simulink model "TST_CrCtl_StTrans"  (R2016b)
settings: Solver=FixedStepDiscrete  StartTime=0.0  StopTime=simTime  FixedStep=sampleTime  RelTol=1e-3
values from neighbouring files (symbols this model uses):
  testCase = 1    [initTST_CrCtl_StTrans_001.m]    (also in initTST_CrCtl_StTrans_002.m = 2; initTST_CrCtl_StTrans_003.m = 3; initTST_CrCtl_StTrans_004.m = 4; initTST_CrCtl_StTrans_005.m = 5)
libraries: simulink x46, UnitTest_Lib x5
(part 2 of 2)

== system TST_CrCtl_StTrans/simulationInput/testSignals_R003 ==
  BC : BusCreator  Inputs=22
  spec_CrCUI_stBttn : FromWorkspace  VariableName=testSig_CrCUI_stBttn  Interpolate=off  OutputAfterFinalValue=Holding final value
  spec_CrCtl_rTraV2NBeg : FromWorkspace  VariableName=testSig_CrCtl_rTraV2NBeg  Interpolate=off  OutputAfterFinalValue=Holding final value
  spec_CrCtl_rTraV2NBeg_raw : FromWorkspace  VariableName=testSig_CrCtl_rTraV2NBeg_raw  Interpolate=off  OutputAfterFinalValue=Holding final value
  spec_CrCtl_st : FromWorkspace  VariableName=testSig_CrCtl_st  Interpolate=off  OutputAfterFinalValue=Holding final value
  spec_CrCtl_stAccSave : FromWorkspace  VariableName=testSig_CrCtl_stAccSave  Interpolate=off  OutputAfterFinalValue=Holding final value
  spec_CrCtl_stCrCUIvLimAdj : FromWorkspace  VariableName=testSig_CrCtl_stCrCUIvLimAdj  Interpolate=off  OutputAfterFinalValue=Holding final value
  spec_CrCtl_stDecSave : FromWorkspace  VariableName=testSig_CrCtl_stDecSave  Interpolate=off  OutputAfterFinalValue=Holding final value
  spec_CrCtl_stLck : FromWorkspace  VariableName=testSig_CrCtl_stLck  Interpolate=off  OutputAfterFinalValue=Holding final value
  spec_CrCtl_stOpFunc : FromWorkspace  VariableName=testSig_CrCtl_stOpFunc  Interpolate=off  OutputAfterFinalValue=Holding final value
  spec_CrCtl_stReq : FromWorkspace  VariableName=testSig_CrCtl_stReq  Interpolate=off  OutputAfterFinalValue=Holding final value
  spec_CrCtl_stShOff : FromWorkspace  VariableName=testSig_CrCtl_stShOff  Interpolate=off  OutputAfterFinalValue=Holding final value
  spec_CrCtl_stStTrans : FromWorkspace  VariableName=testSig_CrCtl_stStTrans  Interpolate=off  OutputAfterFinalValue=Holding final value
  spec_CrCtl_stSub : FromWorkspace  VariableName=testSig_CrCtl_stSub  Interpolate=off  OutputAfterFinalValue=Holding final value
  spec_CrCtl_stSub_raw : FromWorkspace  VariableName=testSig_CrCtl_stSub_raw  Interpolate=off  OutputAfterFinalValue=Holding final value
  spec_CrCtl_stSusp : FromWorkspace  VariableName=testSig_CrCtl_stSusp  Interpolate=off  OutputAfterFinalValue=Holding final value
  spec_CrCtl_stSuspAct : FromWorkspace  VariableName=testSig_CrCtl_stSuspAct  Interpolate=off  OutputAfterFinalValue=Holding final value
  spec_CrCtl_st_raw : FromWorkspace  VariableName=testSig_CrCtl_st_raw  Interpolate=off  OutputAfterFinalValue=Holding final value
  spec_CrCtl_vDes : FromWorkspace  VariableName=testSig_CrCtl_vDes  Interpolate=off  OutputAfterFinalValue=Holding final value
  spec_GlbDa_vXFlt : FromWorkspace  VariableName=testSig_GlbDa_vXFlt  Interpolate=off  OutputAfterFinalValue=Holding final value
  spec_LLim_stModify : FromWorkspace  VariableName=testSig_LLim_stModify  Interpolate=off  OutputAfterFinalValue=Holding final value
  spec_PT_rTraV2N : FromWorkspace  VariableName=testSig_PT_rTraV2N  Interpolate=off  OutputAfterFinalValue=Holding final value
  spec_WESDem_stCurr : FromWorkspace  VariableName=testSig_WESDem_stCurr  Interpolate=off  OutputAfterFinalValue=Holding final value
  testSignals : Outport
  wires:
  BC/1 -> testSignals/1
  spec_CrCtl_stLck/1 -> BC/1  "testSig_CrCtl_stLck"
  spec_CrCtl_stOpFunc/1 -> BC/2  "testSig_CrCtl_stOpFunc"
  spec_CrCtl_stReq/1 -> BC/3  "testSig_CrCtl_stReq"
  spec_CrCtl_stShOff/1 -> BC/4  "testSig_CrCtl_stShOff"
  spec_CrCtl_stSuspAct/1 -> BC/5  "testSig_CrCtl_stSuspAct"
  spec_CrCtl_vDes/1 -> BC/6  "testSig_CrCtl_vDes"
  spec_CrCUI_stBttn/1 -> BC/7  "testSig_CrCUI_stBttn"
  spec_GlbDa_vXFlt/1 -> BC/8  "testSig_GlbDa_vXFlt"
  spec_LLim_stModify/1 -> BC/9  "testSig_LLim_stModify"
  spec_PT_rTraV2N/1 -> BC/10  "testSig_PT_rTraV2N"
  spec_WESDem_stCurr/1 -> BC/11  "testSig_WESDem_stCurr"
  spec_CrCtl_st/1 -> BC/12  "testSig_CrCtl_st"
  spec_CrCtl_stSub/1 -> BC/13  "testSig_CrCtl_stSub"
  spec_CrCtl_rTraV2NBeg/1 -> BC/14  "testSig_CrCtl_rTraV2NBeg"
  spec_CrCtl_stAccSave/1 -> BC/15  "testSig_CrCtl_stAccSave"
  spec_CrCtl_stCrCUIvLimAdj/1 -> BC/16  "testSig_CrCtl_stCrCUIvLimAdj"
  spec_CrCtl_stDecSave/1 -> BC/17  "testSig_CrCtl_stDecSave"
  spec_CrCtl_stStTrans/1 -> BC/18  "testSig_CrCtl_stStTrans"
  spec_CrCtl_stSusp/1 -> BC/19  "testSig_CrCtl_stSusp"
  spec_CrCtl_rTraV2NBeg_raw/1 -> BC/20  "testSig_CrCtl_rTraV2NBeg_raw"
  spec_CrCtl_st_raw/1 -> BC/21  "testSig_CrCtl_st_raw"
  spec_CrCtl_stSub_raw/1 -> BC/22  "testSig_CrCtl_stSub_raw"

== system TST_CrCtl_StTrans/simulationInput/testSignals_R004 ==
  BC : BusCreator  Inputs=22
  spec_CrCUI_stBttn : FromWorkspace  VariableName=testSig_CrCUI_stBttn  Interpolate=off  OutputAfterFinalValue=Holding final value
  spec_CrCtl_rTraV2NBeg : FromWorkspace  VariableName=testSig_CrCtl_rTraV2NBeg  Interpolate=off  OutputAfterFinalValue=Holding final value
  spec_CrCtl_rTraV2NBeg_raw : FromWorkspace  VariableName=testSig_CrCtl_rTraV2NBeg_raw  Interpolate=off  OutputAfterFinalValue=Holding final value
  spec_CrCtl_st : FromWorkspace  VariableName=testSig_CrCtl_st  Interpolate=off  OutputAfterFinalValue=Holding final value
  spec_CrCtl_stAccSave : FromWorkspace  VariableName=testSig_CrCtl_stAccSave  Interpolate=off  OutputAfterFinalValue=Holding final value
  spec_CrCtl_stCrCUIvLimAdj : FromWorkspace  VariableName=testSig_CrCtl_stCrCUIvLimAdj  Interpolate=off  OutputAfterFinalValue=Holding final value
  spec_CrCtl_stDecSave : FromWorkspace  VariableName=testSig_CrCtl_stDecSave  Interpolate=off  OutputAfterFinalValue=Holding final value
  spec_CrCtl_stLck : FromWorkspace  VariableName=testSig_CrCtl_stLck  Interpolate=off  OutputAfterFinalValue=Holding final value
  spec_CrCtl_stOpFunc : FromWorkspace  VariableName=testSig_CrCtl_stOpFunc  Interpolate=off  OutputAfterFinalValue=Holding final value
  spec_CrCtl_stReq : FromWorkspace  VariableName=testSig_CrCtl_stReq  Interpolate=off  OutputAfterFinalValue=Holding final value
  spec_CrCtl_stShOff : FromWorkspace  VariableName=testSig_CrCtl_stShOff  Interpolate=off  OutputAfterFinalValue=Holding final value
  spec_CrCtl_stStTrans : FromWorkspace  VariableName=testSig_CrCtl_stStTrans  Interpolate=off  OutputAfterFinalValue=Holding final value
  spec_CrCtl_stSub : FromWorkspace  VariableName=testSig_CrCtl_stSub  Interpolate=off  OutputAfterFinalValue=Holding final value
  spec_CrCtl_stSub_raw : FromWorkspace  VariableName=testSig_CrCtl_stSub_raw  Interpolate=off  OutputAfterFinalValue=Holding final value
  spec_CrCtl_stSusp : FromWorkspace  VariableName=testSig_CrCtl_stSusp  Interpolate=off  OutputAfterFinalValue=Holding final value
  spec_CrCtl_stSuspAct : FromWorkspace  VariableName=testSig_CrCtl_stSuspAct  Interpolate=off  OutputAfterFinalValue=Holding final value
  spec_CrCtl_st_raw : FromWorkspace  VariableName=testSig_CrCtl_st_raw  Interpolate=off  OutputAfterFinalValue=Holding final value
  spec_CrCtl_vDes : FromWorkspace  VariableName=testSig_CrCtl_vDes  Interpolate=off  OutputAfterFinalValue=Holding final value
  spec_GlbDa_vXFlt : FromWorkspace  VariableName=testSig_GlbDa_vXFlt  Interpolate=off  OutputAfterFinalValue=Holding final value
  spec_LLim_stModify : FromWorkspace  VariableName=testSig_LLim_stModify  Interpolate=off  OutputAfterFinalValue=Holding final value
  spec_PT_rTraV2N : FromWorkspace  VariableName=testSig_PT_rTraV2N  Interpolate=off  OutputAfterFinalValue=Holding final value
  spec_WESDem_stCurr : FromWorkspace  VariableName=testSig_WESDem_stCurr  Interpolate=off  OutputAfterFinalValue=Holding final value
  testSignals : Outport
  wires:
  BC/1 -> testSignals/1
  spec_CrCtl_stLck/1 -> BC/1  "testSig_CrCtl_stLck"
  spec_CrCtl_stOpFunc/1 -> BC/2  "testSig_CrCtl_stOpFunc"
  spec_CrCtl_stReq/1 -> BC/3  "testSig_CrCtl_stReq"
  spec_CrCtl_stShOff/1 -> BC/4  "testSig_CrCtl_stShOff"
  spec_CrCtl_stSuspAct/1 -> BC/5  "testSig_CrCtl_stSuspAct"
  spec_CrCtl_vDes/1 -> BC/6  "testSig_CrCtl_vDes"
  spec_CrCUI_stBttn/1 -> BC/7  "testSig_CrCUI_stBttn"
  spec_GlbDa_vXFlt/1 -> BC/8  "testSig_GlbDa_vXFlt"
  spec_LLim_stModify/1 -> BC/9  "testSig_LLim_stModify"
  spec_PT_rTraV2N/1 -> BC/10  "testSig_PT_rTraV2N"
  spec_WESDem_stCurr/1 -> BC/11  "testSig_WESDem_stCurr"
  spec_CrCtl_st/1 -> BC/12  "testSig_CrCtl_st"
  spec_CrCtl_stSub/1 -> BC/13  "testSig_CrCtl_stSub"
  spec_CrCtl_rTraV2NBeg/1 -> BC/14  "testSig_CrCtl_rTraV2NBeg"
  spec_CrCtl_stAccSave/1 -> BC/15  "testSig_CrCtl_stAccSave"
  spec_CrCtl_stCrCUIvLimAdj/1 -> BC/16  "testSig_CrCtl_stCrCUIvLimAdj"
  spec_CrCtl_stDecSave/1 -> BC/17  "testSig_CrCtl_stDecSave"
  spec_CrCtl_stStTrans/1 -> BC/18  "testSig_CrCtl_stStTrans"
  spec_CrCtl_stSusp/1 -> BC/19  "testSig_CrCtl_stSusp"
  spec_CrCtl_rTraV2NBeg_raw/1 -> BC/20  "testSig_CrCtl_rTraV2NBeg_raw"
  spec_CrCtl_st_raw/1 -> BC/21  "testSig_CrCtl_st_raw"
  spec_CrCtl_stSub_raw/1 -> BC/22  "testSig_CrCtl_stSub_raw"

== system TST_CrCtl_StTrans/simulationInput/testSignals_R005 ==
  BC : BusCreator  Inputs=22
  spec_CrCUI_stBttn : FromWorkspace  VariableName=testSig_CrCUI_stBttn  Interpolate=off  OutputAfterFinalValue=Holding final value
  spec_CrCtl_rTraV2NBeg : FromWorkspace  VariableName=testSig_CrCtl_rTraV2NBeg  Interpolate=off  OutputAfterFinalValue=Holding final value
  spec_CrCtl_rTraV2NBeg_raw : FromWorkspace  VariableName=testSig_CrCtl_rTraV2NBeg_raw  Interpolate=off  OutputAfterFinalValue=Holding final value
  spec_CrCtl_st : FromWorkspace  VariableName=testSig_CrCtl_st  Interpolate=off  OutputAfterFinalValue=Holding final value
  spec_CrCtl_stAccSave : FromWorkspace  VariableName=testSig_CrCtl_stAccSave  Interpolate=off  OutputAfterFinalValue=Holding final value
  spec_CrCtl_stCrCUIvLimAdj : FromWorkspace  VariableName=testSig_CrCtl_stCrCUIvLimAdj  Interpolate=off  OutputAfterFinalValue=Holding final value
  spec_CrCtl_stDecSave : FromWorkspace  VariableName=testSig_CrCtl_stDecSave  Interpolate=off  OutputAfterFinalValue=Holding final value
  spec_CrCtl_stLck : FromWorkspace  VariableName=testSig_CrCtl_stLck  Interpolate=off  OutputAfterFinalValue=Holding final value
  spec_CrCtl_stOpFunc : FromWorkspace  VariableName=testSig_CrCtl_stOpFunc  Interpolate=off  OutputAfterFinalValue=Holding final value
  spec_CrCtl_stReq : FromWorkspace  VariableName=testSig_CrCtl_stReq  Interpolate=off  OutputAfterFinalValue=Holding final value
  spec_CrCtl_stShOff : FromWorkspace  VariableName=testSig_CrCtl_stShOff  Interpolate=off  OutputAfterFinalValue=Holding final value
  spec_CrCtl_stStTrans : FromWorkspace  VariableName=testSig_CrCtl_stStTrans  Interpolate=off  OutputAfterFinalValue=Holding final value
  spec_CrCtl_stSub : FromWorkspace  VariableName=testSig_CrCtl_stSub  Interpolate=off  OutputAfterFinalValue=Holding final value
  spec_CrCtl_stSub_raw : FromWorkspace  VariableName=testSig_CrCtl_stSub_raw  Interpolate=off  OutputAfterFinalValue=Holding final value
  spec_CrCtl_stSusp : FromWorkspace  VariableName=testSig_CrCtl_stSusp  Interpolate=off  OutputAfterFinalValue=Holding final value
  spec_CrCtl_stSuspAct : FromWorkspace  VariableName=testSig_CrCtl_stSuspAct  Interpolate=off  OutputAfterFinalValue=Holding final value
  spec_CrCtl_st_raw : FromWorkspace  VariableName=testSig_CrCtl_st_raw  Interpolate=off  OutputAfterFinalValue=Holding final value
  spec_CrCtl_vDes : FromWorkspace  VariableName=testSig_CrCtl_vDes  Interpolate=off  OutputAfterFinalValue=Holding final value
  spec_GlbDa_vXFlt : FromWorkspace  VariableName=testSig_GlbDa_vXFlt  Interpolate=off  OutputAfterFinalValue=Holding final value
  spec_LLim_stModify : FromWorkspace  VariableName=testSig_LLim_stModify  Interpolate=off  OutputAfterFinalValue=Holding final value
  spec_PT_rTraV2N : FromWorkspace  VariableName=testSig_PT_rTraV2N  Interpolate=off  OutputAfterFinalValue=Holding final value
  spec_WESDem_stCurr : FromWorkspace  VariableName=testSig_WESDem_stCurr  Interpolate=off  OutputAfterFinalValue=Holding final value
  testSignals : Outport
  wires:
  BC/1 -> testSignals/1
  spec_CrCtl_stLck/1 -> BC/1  "testSig_CrCtl_stLck"
  spec_CrCtl_stOpFunc/1 -> BC/2  "testSig_CrCtl_stOpFunc"
  spec_CrCtl_stReq/1 -> BC/3  "testSig_CrCtl_stReq"
  spec_CrCtl_stShOff/1 -> BC/4  "testSig_CrCtl_stShOff"
  spec_CrCtl_stSuspAct/1 -> BC/5  "testSig_CrCtl_stSuspAct"
  spec_CrCtl_vDes/1 -> BC/6  "testSig_CrCtl_vDes"
  spec_CrCUI_stBttn/1 -> BC/7  "testSig_CrCUI_stBttn"
  spec_GlbDa_vXFlt/1 -> BC/8  "testSig_GlbDa_vXFlt"
  spec_LLim_stModify/1 -> BC/9  "testSig_LLim_stModify"
  spec_PT_rTraV2N/1 -> BC/10  "testSig_PT_rTraV2N"
  spec_WESDem_stCurr/1 -> BC/11  "testSig_WESDem_stCurr"
  spec_CrCtl_st/1 -> BC/12  "testSig_CrCtl_st"
  spec_CrCtl_stSub/1 -> BC/13  "testSig_CrCtl_stSub"
  spec_CrCtl_rTraV2NBeg/1 -> BC/14  "testSig_CrCtl_rTraV2NBeg"
  spec_CrCtl_stAccSave/1 -> BC/15  "testSig_CrCtl_stAccSave"
  spec_CrCtl_stCrCUIvLimAdj/1 -> BC/16  "testSig_CrCtl_stCrCUIvLimAdj"
  spec_CrCtl_stDecSave/1 -> BC/17  "testSig_CrCtl_stDecSave"
  spec_CrCtl_stStTrans/1 -> BC/18  "testSig_CrCtl_stStTrans"
  spec_CrCtl_stSusp/1 -> BC/19  "testSig_CrCtl_stSusp"
  spec_CrCtl_rTraV2NBeg_raw/1 -> BC/20  "testSig_CrCtl_rTraV2NBeg_raw"
  spec_CrCtl_st_raw/1 -> BC/21  "testSig_CrCtl_st_raw"
  spec_CrCtl_stSub_raw/1 -> BC/22  "testSig_CrCtl_stSub_raw"

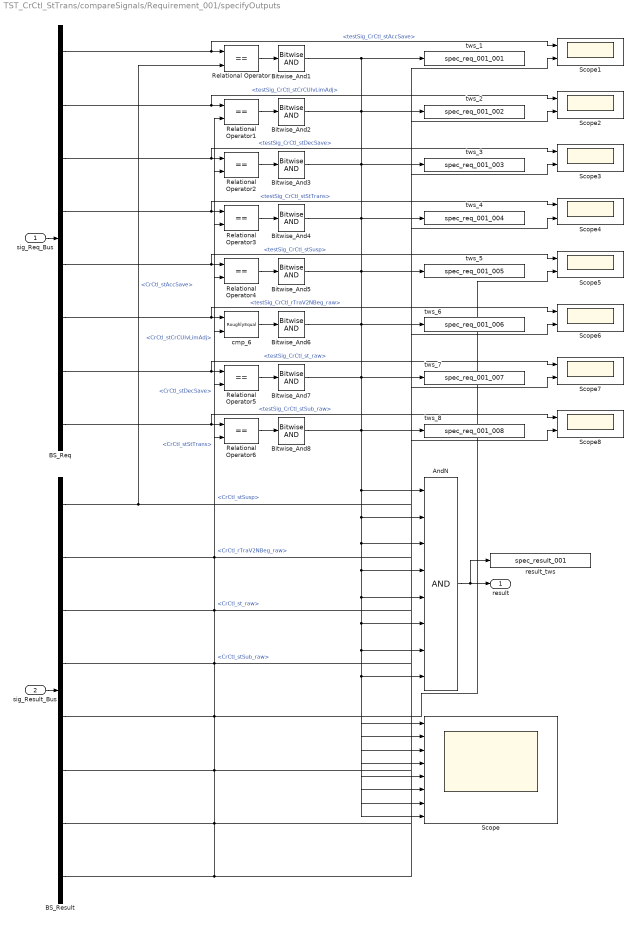
== system TST_CrCtl_StTrans/compareSignals/Requirement_001/specifyOutputs ==
  sig_Req_Bus : Inport
  sig_Result_Bus : Inport  Port=2
  AndN : Logic  Inputs=8
  BS_Req : BusSelector  OutputSignals=testSig_CrCtl_stAccSave,testSig_CrCtl_stCrCUIvLimAdj,testSig_CrCtl_stDecSave,testSig_CrCtl_stStTrans,testSig_CrCtl_stSusp,testSig_CrCtl_rTraV2NBeg_raw,testSig_CrCtl_st_raw,testSig_CrCtl_stSub_raw
  BS_Result : BusSelector  OutputSignals=CrCtl_stAccSave,CrCtl_stCrCUIvLimAdj,CrCtl_stDecSave,CrCtl_stStTrans,CrCtl_stSusp,CrCtl_rTraV2NBeg_raw,CrCtl_st_raw,CrCtl_stSub_raw
  Bitwise_And{1..8} (8 alike) : simulink/Logic and Bit Operations/Bitwise Operator  logicop=AND  UseBitMask=off  BitMask=bin2dec('11011001')  BitMaskRealWorld=Stored Integer
  Relational Operator{,1..6} (7 alike) : RelationalOperator  Operator===  OutDataTypeStr=boolean  RndMeth=Simplest
  Scope : Scope  NumInputPorts=8
  Scope{1..8} (8 alike) : Scope  NumInputPorts=2
  cmp_6 : UnitTest_Lib/RoughlyEqual  slope=0.1
  result_tws : ToWorkspace  VariableName=spec_result_001
  tws_1 : ToWorkspace  VariableName=spec_req_001_001
  tws_2 : ToWorkspace  VariableName=spec_req_001_002
  tws_3 : ToWorkspace  VariableName=spec_req_001_003
  tws_4 : ToWorkspace  VariableName=spec_req_001_004
  tws_5 : ToWorkspace  VariableName=spec_req_001_005
  tws_6 : ToWorkspace  VariableName=spec_req_001_006
  tws_7 : ToWorkspace  VariableName=spec_req_001_007
  tws_8 : ToWorkspace  VariableName=spec_req_001_008
  result : Outport
  wires:
  sig_Req_Bus/1 -> BS_Req/1
  sig_Result_Bus/1 -> BS_Result/1
  AndN/1 -> result/1, result_tws/1
  BS_Req/1 -> Relational Operator/1, Scope1/1  "<testSig_CrCtl_stAccSave>"
  BS_Result/1 -> Relational Operator/2, Scope1/2  "<CrCtl_stAccSave>"
  Relational Operator/1 -> Bitwise_And1/1
  Bitwise_And1/1 -> AndN/1, Scope/1, tws_1/1
  BS_Req/2 -> Relational Operator1/1, Scope2/1  "<testSig_CrCtl_stCrCUIvLimAdj>"
  BS_Result/2 -> Relational Operator1/2, Scope2/2  "<CrCtl_stCrCUIvLimAdj>"
  Relational Operator1/1 -> Bitwise_And2/1
  Bitwise_And2/1 -> AndN/2, Scope/2, tws_2/1
  BS_Req/3 -> Relational Operator2/1, Scope3/1  "<testSig_CrCtl_stDecSave>"
  BS_Result/3 -> Relational Operator2/2, Scope3/2  "<CrCtl_stDecSave>"
  Relational Operator2/1 -> Bitwise_And3/1
  Bitwise_And3/1 -> AndN/3, Scope/3, tws_3/1
  BS_Req/4 -> Relational Operator3/1, Scope4/1  "<testSig_CrCtl_stStTrans>"
  BS_Result/4 -> Relational Operator3/2, Scope4/2  "<CrCtl_stStTrans>"
  Relational Operator3/1 -> Bitwise_And4/1
  Bitwise_And4/1 -> AndN/4, Scope/4, tws_4/1
  BS_Req/5 -> Relational Operator4/1, Scope5/1  "<testSig_CrCtl_stSusp>"
  BS_Result/5 -> Relational Operator4/2, Scope5/2  "<CrCtl_stSusp>"
  Relational Operator4/1 -> Bitwise_And5/1
  Bitwise_And5/1 -> AndN/5, Scope/5, tws_5/1
  BS_Req/6 -> cmp_6/1, Scope6/1  "<testSig_CrCtl_rTraV2NBeg_raw>"
  BS_Result/6 -> cmp_6/2, Scope6/2  "<CrCtl_rTraV2NBeg_raw>"
  cmp_6/1 -> Bitwise_And6/1
  Bitwise_And6/1 -> AndN/6, Scope/6, tws_6/1
  BS_Req/7 -> Relational Operator5/1, Scope7/1  "<testSig_CrCtl_st_raw>"
  BS_Result/7 -> Relational Operator5/2, Scope7/2  "<CrCtl_st_raw>"
  Relational Operator5/1 -> Bitwise_And7/1
  Bitwise_And7/1 -> AndN/7, Scope/7, tws_7/1
  BS_Req/8 -> Relational Operator6/1, Scope8/1  "<testSig_CrCtl_stSub_raw>"
  BS_Result/8 -> Relational Operator6/2, Scope8/2  "<CrCtl_stSub_raw>"
  Relational Operator6/1 -> Bitwise_And8/1
  Bitwise_And8/1 -> AndN/8, Scope/8, tws_8/1

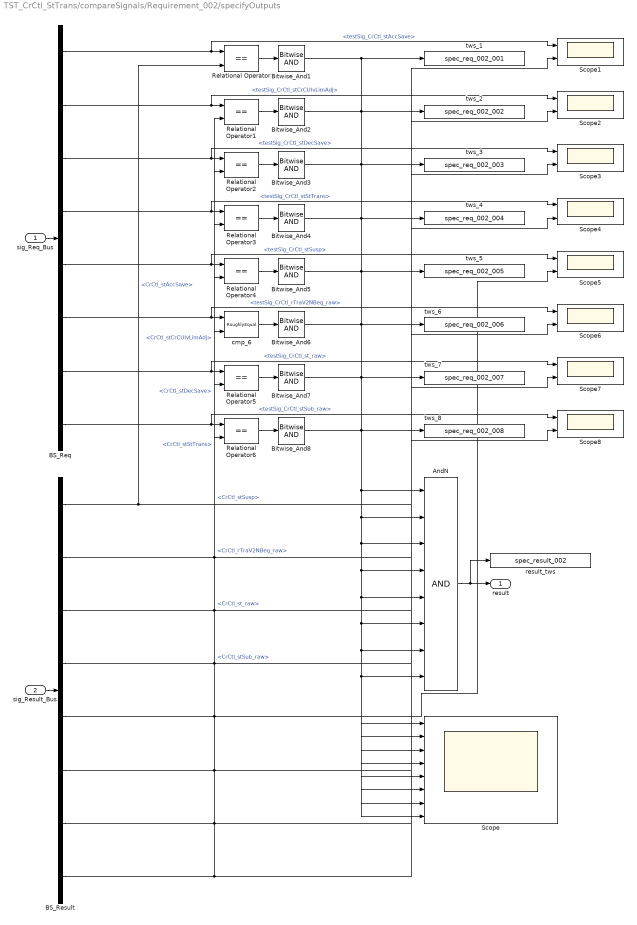
== system TST_CrCtl_StTrans/compareSignals/Requirement_002/specifyOutputs ==
  sig_Req_Bus : Inport
  sig_Result_Bus : Inport  Port=2
  AndN : Logic  Inputs=8
  BS_Req : BusSelector  OutputSignals=testSig_CrCtl_stAccSave,testSig_CrCtl_stCrCUIvLimAdj,testSig_CrCtl_stDecSave,testSig_CrCtl_stStTrans,testSig_CrCtl_stSusp,testSig_CrCtl_rTraV2NBeg_raw,testSig_CrCtl_st_raw,testSig_CrCtl_stSub_raw
  BS_Result : BusSelector  OutputSignals=CrCtl_stAccSave,CrCtl_stCrCUIvLimAdj,CrCtl_stDecSave,CrCtl_stStTrans,CrCtl_stSusp,CrCtl_rTraV2NBeg_raw,CrCtl_st_raw,CrCtl_stSub_raw
  Bitwise_And{1..8} (8 alike) : simulink/Logic and Bit Operations/Bitwise Operator  logicop=AND  UseBitMask=off  BitMask=bin2dec('11011001')  BitMaskRealWorld=Stored Integer
  Relational Operator{,1..6} (7 alike) : RelationalOperator  Operator===  OutDataTypeStr=boolean  RndMeth=Simplest
  Scope : Scope  NumInputPorts=8
  Scope{1..8} (8 alike) : Scope  NumInputPorts=2
  cmp_6 : UnitTest_Lib/RoughlyEqual  slope=0.1
  result_tws : ToWorkspace  VariableName=spec_result_002
  tws_1 : ToWorkspace  VariableName=spec_req_002_001
  tws_2 : ToWorkspace  VariableName=spec_req_002_002
  tws_3 : ToWorkspace  VariableName=spec_req_002_003
  tws_4 : ToWorkspace  VariableName=spec_req_002_004
  tws_5 : ToWorkspace  VariableName=spec_req_002_005
  tws_6 : ToWorkspace  VariableName=spec_req_002_006
  tws_7 : ToWorkspace  VariableName=spec_req_002_007
  tws_8 : ToWorkspace  VariableName=spec_req_002_008
  result : Outport
  wires:
  sig_Req_Bus/1 -> BS_Req/1
  sig_Result_Bus/1 -> BS_Result/1
  AndN/1 -> result/1, result_tws/1
  BS_Req/1 -> Relational Operator/1, Scope1/1  "<testSig_CrCtl_stAccSave>"
  BS_Result/1 -> Relational Operator/2, Scope1/2  "<CrCtl_stAccSave>"
  Relational Operator/1 -> Bitwise_And1/1
  Bitwise_And1/1 -> AndN/1, Scope/1, tws_1/1
  BS_Req/2 -> Relational Operator1/1, Scope2/1  "<testSig_CrCtl_stCrCUIvLimAdj>"
  BS_Result/2 -> Relational Operator1/2, Scope2/2  "<CrCtl_stCrCUIvLimAdj>"
  Relational Operator1/1 -> Bitwise_And2/1
  Bitwise_And2/1 -> AndN/2, Scope/2, tws_2/1
  BS_Req/3 -> Relational Operator2/1, Scope3/1  "<testSig_CrCtl_stDecSave>"
  BS_Result/3 -> Relational Operator2/2, Scope3/2  "<CrCtl_stDecSave>"
  Relational Operator2/1 -> Bitwise_And3/1
  Bitwise_And3/1 -> AndN/3, Scope/3, tws_3/1
  BS_Req/4 -> Relational Operator3/1, Scope4/1  "<testSig_CrCtl_stStTrans>"
  BS_Result/4 -> Relational Operator3/2, Scope4/2  "<CrCtl_stStTrans>"
  Relational Operator3/1 -> Bitwise_And4/1
  Bitwise_And4/1 -> AndN/4, Scope/4, tws_4/1
  BS_Req/5 -> Relational Operator4/1, Scope5/1  "<testSig_CrCtl_stSusp>"
  BS_Result/5 -> Relational Operator4/2, Scope5/2  "<CrCtl_stSusp>"
  Relational Operator4/1 -> Bitwise_And5/1
  Bitwise_And5/1 -> AndN/5, Scope/5, tws_5/1
  BS_Req/6 -> cmp_6/1, Scope6/1  "<testSig_CrCtl_rTraV2NBeg_raw>"
  BS_Result/6 -> cmp_6/2, Scope6/2  "<CrCtl_rTraV2NBeg_raw>"
  cmp_6/1 -> Bitwise_And6/1
  Bitwise_And6/1 -> AndN/6, Scope/6, tws_6/1
  BS_Req/7 -> Relational Operator5/1, Scope7/1  "<testSig_CrCtl_st_raw>"
  BS_Result/7 -> Relational Operator5/2, Scope7/2  "<CrCtl_st_raw>"
  Relational Operator5/1 -> Bitwise_And7/1
  Bitwise_And7/1 -> AndN/7, Scope/7, tws_7/1
  BS_Req/8 -> Relational Operator6/1, Scope8/1  "<testSig_CrCtl_stSub_raw>"
  BS_Result/8 -> Relational Operator6/2, Scope8/2  "<CrCtl_stSub_raw>"
  Relational Operator6/1 -> Bitwise_And8/1
  Bitwise_And8/1 -> AndN/8, Scope/8, tws_8/1

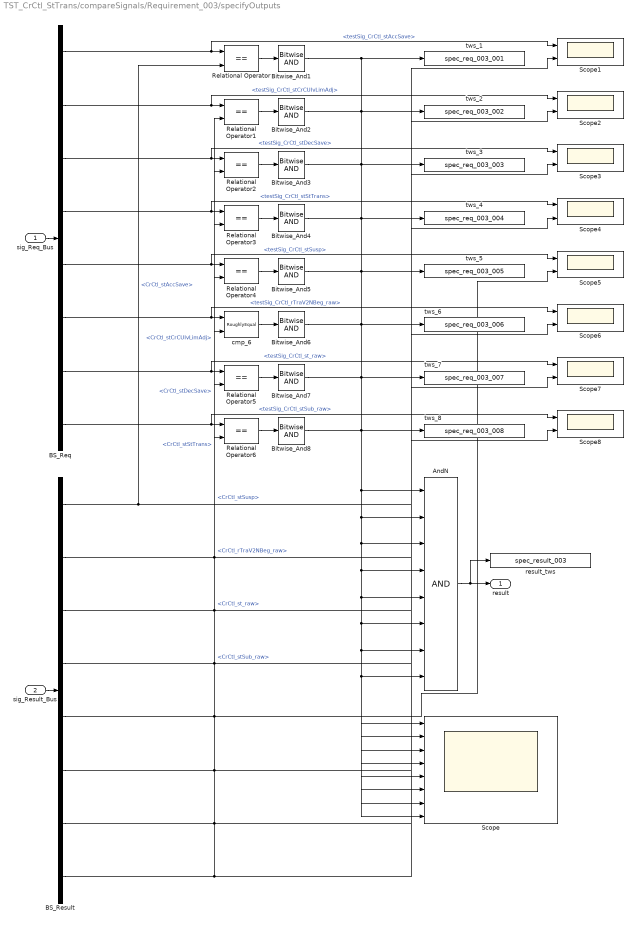
== system TST_CrCtl_StTrans/compareSignals/Requirement_003/specifyOutputs ==
  sig_Req_Bus : Inport
  sig_Result_Bus : Inport  Port=2
  AndN : Logic  Inputs=8
  BS_Req : BusSelector  OutputSignals=testSig_CrCtl_stAccSave,testSig_CrCtl_stCrCUIvLimAdj,testSig_CrCtl_stDecSave,testSig_CrCtl_stStTrans,testSig_CrCtl_stSusp,testSig_CrCtl_rTraV2NBeg_raw,testSig_CrCtl_st_raw,testSig_CrCtl_stSub_raw
  BS_Result : BusSelector  OutputSignals=CrCtl_stAccSave,CrCtl_stCrCUIvLimAdj,CrCtl_stDecSave,CrCtl_stStTrans,CrCtl_stSusp,CrCtl_rTraV2NBeg_raw,CrCtl_st_raw,CrCtl_stSub_raw
  Bitwise_And{1..8} (8 alike) : simulink/Logic and Bit Operations/Bitwise Operator  logicop=AND  UseBitMask=off  BitMask=bin2dec('11011001')  BitMaskRealWorld=Stored Integer
  Relational Operator{,1..6} (7 alike) : RelationalOperator  Operator===  OutDataTypeStr=boolean  RndMeth=Simplest
  Scope : Scope  NumInputPorts=8
  Scope{1..8} (8 alike) : Scope  NumInputPorts=2
  cmp_6 : UnitTest_Lib/RoughlyEqual  slope=0.1
  result_tws : ToWorkspace  VariableName=spec_result_003
  tws_1 : ToWorkspace  VariableName=spec_req_003_001
  tws_2 : ToWorkspace  VariableName=spec_req_003_002
  tws_3 : ToWorkspace  VariableName=spec_req_003_003
  tws_4 : ToWorkspace  VariableName=spec_req_003_004
  tws_5 : ToWorkspace  VariableName=spec_req_003_005
  tws_6 : ToWorkspace  VariableName=spec_req_003_006
  tws_7 : ToWorkspace  VariableName=spec_req_003_007
  tws_8 : ToWorkspace  VariableName=spec_req_003_008
  result : Outport
  wires:
  sig_Req_Bus/1 -> BS_Req/1
  sig_Result_Bus/1 -> BS_Result/1
  AndN/1 -> result/1, result_tws/1
  BS_Req/1 -> Relational Operator/1, Scope1/1  "<testSig_CrCtl_stAccSave>"
  BS_Result/1 -> Relational Operator/2, Scope1/2  "<CrCtl_stAccSave>"
  Relational Operator/1 -> Bitwise_And1/1
  Bitwise_And1/1 -> AndN/1, Scope/1, tws_1/1
  BS_Req/2 -> Relational Operator1/1, Scope2/1  "<testSig_CrCtl_stCrCUIvLimAdj>"
  BS_Result/2 -> Relational Operator1/2, Scope2/2  "<CrCtl_stCrCUIvLimAdj>"
  Relational Operator1/1 -> Bitwise_And2/1
  Bitwise_And2/1 -> AndN/2, Scope/2, tws_2/1
  BS_Req/3 -> Relational Operator2/1, Scope3/1  "<testSig_CrCtl_stDecSave>"
  BS_Result/3 -> Relational Operator2/2, Scope3/2  "<CrCtl_stDecSave>"
  Relational Operator2/1 -> Bitwise_And3/1
  Bitwise_And3/1 -> AndN/3, Scope/3, tws_3/1
  BS_Req/4 -> Relational Operator3/1, Scope4/1  "<testSig_CrCtl_stStTrans>"
  BS_Result/4 -> Relational Operator3/2, Scope4/2  "<CrCtl_stStTrans>"
  Relational Operator3/1 -> Bitwise_And4/1
  Bitwise_And4/1 -> AndN/4, Scope/4, tws_4/1
  BS_Req/5 -> Relational Operator4/1, Scope5/1  "<testSig_CrCtl_stSusp>"
  BS_Result/5 -> Relational Operator4/2, Scope5/2  "<CrCtl_stSusp>"
  Relational Operator4/1 -> Bitwise_And5/1
  Bitwise_And5/1 -> AndN/5, Scope/5, tws_5/1
  BS_Req/6 -> cmp_6/1, Scope6/1  "<testSig_CrCtl_rTraV2NBeg_raw>"
  BS_Result/6 -> cmp_6/2, Scope6/2  "<CrCtl_rTraV2NBeg_raw>"
  cmp_6/1 -> Bitwise_And6/1
  Bitwise_And6/1 -> AndN/6, Scope/6, tws_6/1
  BS_Req/7 -> Relational Operator5/1, Scope7/1  "<testSig_CrCtl_st_raw>"
  BS_Result/7 -> Relational Operator5/2, Scope7/2  "<CrCtl_st_raw>"
  Relational Operator5/1 -> Bitwise_And7/1
  Bitwise_And7/1 -> AndN/7, Scope/7, tws_7/1
  BS_Req/8 -> Relational Operator6/1, Scope8/1  "<testSig_CrCtl_stSub_raw>"
  BS_Result/8 -> Relational Operator6/2, Scope8/2  "<CrCtl_stSub_raw>"
  Relational Operator6/1 -> Bitwise_And8/1
  Bitwise_And8/1 -> AndN/8, Scope/8, tws_8/1

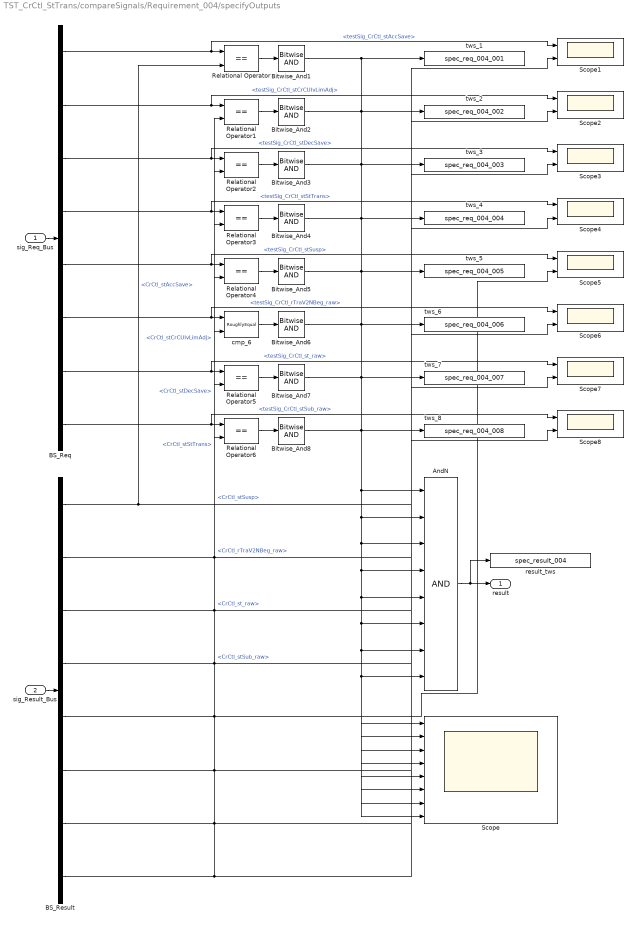
== system TST_CrCtl_StTrans/compareSignals/Requirement_004/specifyOutputs ==
  sig_Req_Bus : Inport
  sig_Result_Bus : Inport  Port=2
  AndN : Logic  Inputs=8
  BS_Req : BusSelector  OutputSignals=testSig_CrCtl_stAccSave,testSig_CrCtl_stCrCUIvLimAdj,testSig_CrCtl_stDecSave,testSig_CrCtl_stStTrans,testSig_CrCtl_stSusp,testSig_CrCtl_rTraV2NBeg_raw,testSig_CrCtl_st_raw,testSig_CrCtl_stSub_raw
  BS_Result : BusSelector  OutputSignals=CrCtl_stAccSave,CrCtl_stCrCUIvLimAdj,CrCtl_stDecSave,CrCtl_stStTrans,CrCtl_stSusp,CrCtl_rTraV2NBeg_raw,CrCtl_st_raw,CrCtl_stSub_raw
  Bitwise_And{1..8} (8 alike) : simulink/Logic and Bit Operations/Bitwise Operator  logicop=AND  UseBitMask=off  BitMask=bin2dec('11011001')  BitMaskRealWorld=Stored Integer
  Relational Operator{,1..6} (7 alike) : RelationalOperator  Operator===  OutDataTypeStr=boolean  RndMeth=Simplest
  Scope : Scope  NumInputPorts=8
  Scope{1..8} (8 alike) : Scope  NumInputPorts=2
  cmp_6 : UnitTest_Lib/RoughlyEqual  slope=0.1
  result_tws : ToWorkspace  VariableName=spec_result_004
  tws_1 : ToWorkspace  VariableName=spec_req_004_001
  tws_2 : ToWorkspace  VariableName=spec_req_004_002
  tws_3 : ToWorkspace  VariableName=spec_req_004_003
  tws_4 : ToWorkspace  VariableName=spec_req_004_004
  tws_5 : ToWorkspace  VariableName=spec_req_004_005
  tws_6 : ToWorkspace  VariableName=spec_req_004_006
  tws_7 : ToWorkspace  VariableName=spec_req_004_007
  tws_8 : ToWorkspace  VariableName=spec_req_004_008
  result : Outport
  wires:
  sig_Req_Bus/1 -> BS_Req/1
  sig_Result_Bus/1 -> BS_Result/1
  AndN/1 -> result/1, result_tws/1
  BS_Req/1 -> Relational Operator/1, Scope1/1  "<testSig_CrCtl_stAccSave>"
  BS_Result/1 -> Relational Operator/2, Scope1/2  "<CrCtl_stAccSave>"
  Relational Operator/1 -> Bitwise_And1/1
  Bitwise_And1/1 -> AndN/1, Scope/1, tws_1/1
  BS_Req/2 -> Relational Operator1/1, Scope2/1  "<testSig_CrCtl_stCrCUIvLimAdj>"
  BS_Result/2 -> Relational Operator1/2, Scope2/2  "<CrCtl_stCrCUIvLimAdj>"
  Relational Operator1/1 -> Bitwise_And2/1
  Bitwise_And2/1 -> AndN/2, Scope/2, tws_2/1
  BS_Req/3 -> Relational Operator2/1, Scope3/1  "<testSig_CrCtl_stDecSave>"
  BS_Result/3 -> Relational Operator2/2, Scope3/2  "<CrCtl_stDecSave>"
  Relational Operator2/1 -> Bitwise_And3/1
  Bitwise_And3/1 -> AndN/3, Scope/3, tws_3/1
  BS_Req/4 -> Relational Operator3/1, Scope4/1  "<testSig_CrCtl_stStTrans>"
  BS_Result/4 -> Relational Operator3/2, Scope4/2  "<CrCtl_stStTrans>"
  Relational Operator3/1 -> Bitwise_And4/1
  Bitwise_And4/1 -> AndN/4, Scope/4, tws_4/1
  BS_Req/5 -> Relational Operator4/1, Scope5/1  "<testSig_CrCtl_stSusp>"
  BS_Result/5 -> Relational Operator4/2, Scope5/2  "<CrCtl_stSusp>"
  Relational Operator4/1 -> Bitwise_And5/1
  Bitwise_And5/1 -> AndN/5, Scope/5, tws_5/1
  BS_Req/6 -> cmp_6/1, Scope6/1  "<testSig_CrCtl_rTraV2NBeg_raw>"
  BS_Result/6 -> cmp_6/2, Scope6/2  "<CrCtl_rTraV2NBeg_raw>"
  cmp_6/1 -> Bitwise_And6/1
  Bitwise_And6/1 -> AndN/6, Scope/6, tws_6/1
  BS_Req/7 -> Relational Operator5/1, Scope7/1  "<testSig_CrCtl_st_raw>"
  BS_Result/7 -> Relational Operator5/2, Scope7/2  "<CrCtl_st_raw>"
  Relational Operator5/1 -> Bitwise_And7/1
  Bitwise_And7/1 -> AndN/7, Scope/7, tws_7/1
  BS_Req/8 -> Relational Operator6/1, Scope8/1  "<testSig_CrCtl_stSub_raw>"
  BS_Result/8 -> Relational Operator6/2, Scope8/2  "<CrCtl_stSub_raw>"
  Relational Operator6/1 -> Bitwise_And8/1
  Bitwise_And8/1 -> AndN/8, Scope/8, tws_8/1

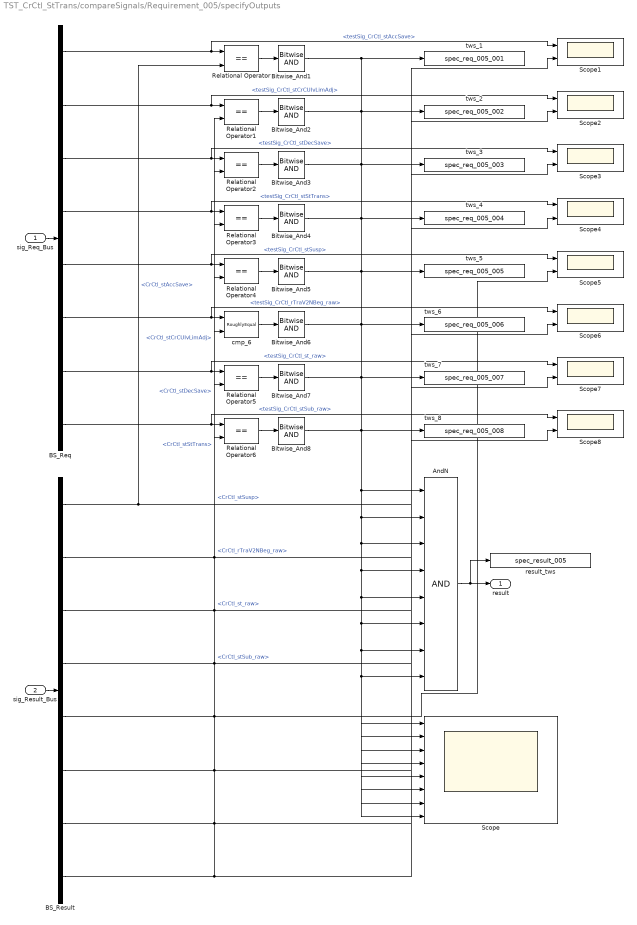
== system TST_CrCtl_StTrans/compareSignals/Requirement_005/specifyOutputs ==
  sig_Req_Bus : Inport
  sig_Result_Bus : Inport  Port=2
  AndN : Logic  Inputs=8
  BS_Req : BusSelector  OutputSignals=testSig_CrCtl_stAccSave,testSig_CrCtl_stCrCUIvLimAdj,testSig_CrCtl_stDecSave,testSig_CrCtl_stStTrans,testSig_CrCtl_stSusp,testSig_CrCtl_rTraV2NBeg_raw,testSig_CrCtl_st_raw,testSig_CrCtl_stSub_raw
  BS_Result : BusSelector  OutputSignals=CrCtl_stAccSave,CrCtl_stCrCUIvLimAdj,CrCtl_stDecSave,CrCtl_stStTrans,CrCtl_stSusp,CrCtl_rTraV2NBeg_raw,CrCtl_st_raw,CrCtl_stSub_raw
  Bitwise_And{1..8} (8 alike) : simulink/Logic and Bit Operations/Bitwise Operator  logicop=AND  UseBitMask=off  BitMask=bin2dec('11011001')  BitMaskRealWorld=Stored Integer
  Relational Operator{,1..6} (7 alike) : RelationalOperator  Operator===  OutDataTypeStr=boolean  RndMeth=Simplest
  Scope : Scope  NumInputPorts=8
  Scope{1..8} (8 alike) : Scope  NumInputPorts=2
  cmp_6 : UnitTest_Lib/RoughlyEqual  slope=0.1
  result_tws : ToWorkspace  VariableName=spec_result_005
  tws_1 : ToWorkspace  VariableName=spec_req_005_001
  tws_2 : ToWorkspace  VariableName=spec_req_005_002
  tws_3 : ToWorkspace  VariableName=spec_req_005_003
  tws_4 : ToWorkspace  VariableName=spec_req_005_004
  tws_5 : ToWorkspace  VariableName=spec_req_005_005
  tws_6 : ToWorkspace  VariableName=spec_req_005_006
  tws_7 : ToWorkspace  VariableName=spec_req_005_007
  tws_8 : ToWorkspace  VariableName=spec_req_005_008
  result : Outport
  wires:
  sig_Req_Bus/1 -> BS_Req/1
  sig_Result_Bus/1 -> BS_Result/1
  AndN/1 -> result/1, result_tws/1
  BS_Req/1 -> Relational Operator/1, Scope1/1  "<testSig_CrCtl_stAccSave>"
  BS_Result/1 -> Relational Operator/2, Scope1/2  "<CrCtl_stAccSave>"
  Relational Operator/1 -> Bitwise_And1/1
  Bitwise_And1/1 -> AndN/1, Scope/1, tws_1/1
  BS_Req/2 -> Relational Operator1/1, Scope2/1  "<testSig_CrCtl_stCrCUIvLimAdj>"
  BS_Result/2 -> Relational Operator1/2, Scope2/2  "<CrCtl_stCrCUIvLimAdj>"
  Relational Operator1/1 -> Bitwise_And2/1
  Bitwise_And2/1 -> AndN/2, Scope/2, tws_2/1
  BS_Req/3 -> Relational Operator2/1, Scope3/1  "<testSig_CrCtl_stDecSave>"
  BS_Result/3 -> Relational Operator2/2, Scope3/2  "<CrCtl_stDecSave>"
  Relational Operator2/1 -> Bitwise_And3/1
  Bitwise_And3/1 -> AndN/3, Scope/3, tws_3/1
  BS_Req/4 -> Relational Operator3/1, Scope4/1  "<testSig_CrCtl_stStTrans>"
  BS_Result/4 -> Relational Operator3/2, Scope4/2  "<CrCtl_stStTrans>"
  Relational Operator3/1 -> Bitwise_And4/1
  Bitwise_And4/1 -> AndN/4, Scope/4, tws_4/1
  BS_Req/5 -> Relational Operator4/1, Scope5/1  "<testSig_CrCtl_stSusp>"
  BS_Result/5 -> Relational Operator4/2, Scope5/2  "<CrCtl_stSusp>"
  Relational Operator4/1 -> Bitwise_And5/1
  Bitwise_And5/1 -> AndN/5, Scope/5, tws_5/1
  BS_Req/6 -> cmp_6/1, Scope6/1  "<testSig_CrCtl_rTraV2NBeg_raw>"
  BS_Result/6 -> cmp_6/2, Scope6/2  "<CrCtl_rTraV2NBeg_raw>"
  cmp_6/1 -> Bitwise_And6/1
  Bitwise_And6/1 -> AndN/6, Scope/6, tws_6/1
  BS_Req/7 -> Relational Operator5/1, Scope7/1  "<testSig_CrCtl_st_raw>"
  BS_Result/7 -> Relational Operator5/2, Scope7/2  "<CrCtl_st_raw>"
  Relational Operator5/1 -> Bitwise_And7/1
  Bitwise_And7/1 -> AndN/7, Scope/7, tws_7/1
  BS_Req/8 -> Relational Operator6/1, Scope8/1  "<testSig_CrCtl_stSub_raw>"
  BS_Result/8 -> Relational Operator6/2, Scope8/2  "<CrCtl_stSub_raw>"
  Relational Operator6/1 -> Bitwise_And8/1
  Bitwise_And8/1 -> AndN/8, Scope/8, tws_8/1
